simulink model "PubIfDecisionLM_MDL"  (R2020b)
settings: configuration reference "DspaceConfig" (kept outside this file)
PostLoadFcn:
  | if any(exist('dsrtsu_mdlpostloadfcn', 'file') ~= 0), dsrtsu_mdlpostloadfcn('Execute', bdroot); end
InitFcn:
  | , if any(exist('dsmpb_private', 'file') ~= 0), dsmpb_private('dsmpb_mdlclblib', 'Init', bdroot); end,
undefined symbols (not defined in the file or in its folder): OFM_OBJ_FUSIONTYPE_E, OFM_OBJ_MOVINGSTATE_E, OFM_OBJ_ORIENTATION_E, OFM_OBJ_TYPE_E, P_LM_Cyc, P_LM_EMLHistKapRcdBufSize, P_LM_EMLHistTrajBaseDis, P_LM_EMLHistTrajPNum, P_LM_EMLKapCorrMaxThre, P_LM_EMLMinKapThre, P_LM_EMLPathDisDiffThre, P_LM_EMLQuaFiltPar, P_LM_EMLTurnActKapThre, P_LM_EMLValidQuaThre, P_LM_FntPath1Disgap, P_LM_FntPath1MinDis, P_LM_FntPath1Timegap, P_LM_FntPath2Disgap, P_LM_FntPath2MinDis, P_LM_FntPath2Timegap, P_LM_FntPath3Disgap, P_LM_FntPath3MinDis, P_LM_FntPath3Timegap, P_LM_FusBLParFiltP, P_LM_FusEVDifC2Thre, P_LM_FusEVOPath1AllVSLDisThre, P_LM_FusEVOPath1AllVSLLostNumThre, P_LM_FusEVOPath1AllVSLQuaThre, P_LM_FusEVOPath1OTLFacNLC, P_LM_FusOTLQuaThre, P_LM_FusOTLSW, P_LM_FusParC0Index, P_LM_FusParC1Index, P_LM_FusParC2Index, P_LM_FusParC3Index, P_LM_FusVSLQuaThre, P_LM_FusVSLSW, P_LM_FusVSLValidSteerWheerAngThre, P_LM_FusVSLValidVxvThre, P_LM_LaneWidth, P_LM_OTLBufTPInfoEvaFactor, P_LM_OTLObjNum, P_LM_OTLObjSelectAgeThre, P_LM_OTLObjSelectDxAssessVx, P_LM_OTLObjSelectDxThre, P_LM_OTLObjSelectVxThre, P_LM_OTLObjSelectVyAssessDx, P_LM_OTLObjSelectVyThre, P_LM_OTLTrajPntBaseDis, P_LM_OTLTrajStdThre, P_LM_VSLAvailLineNum, P_LM_VSLBLSDiffThre, P_LM_VSLBLSDisRatio, P_LM_VSLFusBLParFiltP_C1, P_LM_VSLFusBLParFiltP_C2, P_LM_VSLFusBLParFiltP_C3, P_LM_VSLFusBLParFiltP_Quality, P_LM_VSLHistTrajBaseDis, P_LM_VSLHistTrajPNum, P_LM_VSLLCC0diff ... (+18)
libraries: simulink x145, LM_LIB x43
(part 7 of 24)

== system PubIfDecisionLM_MDL/Subsystem2/LM_EML/LM_EMLFntPath1/LM_EML_C0/Switch Case Action Subsystem1 ==
  P_LM_LaneWidth : Inport
  Action Port : ActionPort  ActionPortLabel=case [ 1 ]:
  Constant : Constant  Value=2  OutDataTypeStr=single
  Constant1 : Constant  Value=-1  OutDataTypeStr=single
  Divide : Product  Inputs=*/
  Product : Product
  Subtract : Sum  Inputs=+-
  Subtract1 : Sum  Inputs=+-
  LM_EML_LLC0 : Outport
  LM_EML_LRC0 : Outport  Port=2
  LM_EML_RLC0 : Outport  Port=3
  LM_EML_RRC0 : Outport  Port=4
  wires:
  Product/1 -> LM_EML_LRC0/1, Subtract1/1  "LM_EML_LRC0"
  Subtract/1 -> LM_EML_RRC0/1  "LM_EML_RRC0"
  P_LM_LaneWidth/1 -> Divide/1, Subtract/2, Subtract1/2
  Constant/1 -> Divide/2
  Subtract1/1 -> LM_EML_RLC0/1, Subtract/1  "LM_EML_RLC0"
  Constant1/1 -> Product/2
  Divide/1 -> LM_EML_LLC0/1, Product/1  "LM_EML_LRC0"

== system PubIfDecisionLM_MDL/Subsystem2/LM_EML/LM_EMLFntPath1/LM_EML_C0/Switch Case Action Subsystem2 ==
  P_LM_LaneWidth : Inport
  Action Port : ActionPort  ActionPortLabel=case [ 3 ]:
  Add : Sum
  Add1 : Sum
  Constant : Constant  Value=2  OutDataTypeStr=single
  Constant1 : Constant  Value=-1  OutDataTypeStr=single
  Divide : Product  Inputs=*/
  Product : Product
  LM_EML_LLC0 : Outport
  LM_EML_LRC0 : Outport  Port=2
  LM_EML_RLC0 : Outport  Port=3
  LM_EML_RRC0 : Outport  Port=4
  wires:
  Add/1 -> LM_EML_LRC0/1, Add1/2  "LM_EML_LRC0"
  Divide/1 -> LM_EML_RLC0/1, Add/2, Product/1  "LM_EML_RLC0"
  Constant1/1 -> Product/2
  Constant/1 -> Divide/2
  P_LM_LaneWidth/1 -> Add1/1, Add/1, Divide/1
  Add1/1 -> LM_EML_LLC0/1  "LM_EML_LLC0"
  Product/1 -> LM_EML_RRC0/1  "LM_EML_RRC0"

== system PubIfDecisionLM_MDL/Subsystem2/LM_EML/LM_EMLRearPath1/LM_EMLHistTrajCoordinateConvert/If Action Subsystem ==
  LM_ComEVOffsetX : Inport
  LM_ComEVOffsetY : Inport  Port=2
  LM_ComEVOffsetAng : Inport  Port=3
  LM_EMLHistTrajVectXK1 : Inport  Port=4
  LM_EMLHistTrajVectYK1 : Inport  Port=5
  Action Port : ActionPort  ActionPortLabel=if(u1 == 0)
  For Each Subsystem : Subsystem  TreatAsAtomicUnit=on
  LM_EMLHistTrajVectXK1Adju : Outport
  LM_EMLHistTrajVectYK1Adju : Outport  Port=2
  wires:
  For Each Subsystem/2(LM_EMLHistTrajVectYK1Adju) -> LM_EMLHistTrajVectYK1Adju/1
  For Each Subsystem/1(LM_EMLHistTrajVectXK1Adju) -> LM_EMLHistTrajVectXK1Adju/1
  LM_EMLHistTrajVectYK1/1 -> For Each Subsystem/5(LM_EMLHistTrajVectYK1)
  LM_EMLHistTrajVectXK1/1 -> For Each Subsystem/4(LM_EMLHistTrajVectXK1)
  LM_ComEVOffsetAng/1 -> For Each Subsystem/3(LM_ComEVOffsetAng)
  LM_ComEVOffsetY/1 -> For Each Subsystem/2(LM_ComEVOffsetY)
  LM_ComEVOffsetX/1 -> For Each Subsystem/1(LM_ComEVOffsetX)

== system PubIfDecisionLM_MDL/Subsystem2/LM_EML/LM_EMLRearPath1/LM_EMLHistTrajCoordinateConvert/If Action Subsystem1 ==
  LM_EMLHistTrajVectXK1 : Inport
  LM_EMLHistTrajVectYK1 : Inport  Port=2
  Action Port : ActionPort  ActionPortLabel=else
  LM_EMLHistTrajVectXK1Adju : Outport
  LM_EMLHistTrajVectYK1Adju : Outport  Port=2
  wires:
  LM_EMLHistTrajVectYK1/1 -> LM_EMLHistTrajVectYK1Adju/1
  LM_EMLHistTrajVectXK1/1 -> LM_EMLHistTrajVectXK1Adju/1

== system PubIfDecisionLM_MDL/Subsystem2/LM_Fusion1/LM_FusBaseLineFilt/LM_FusBaseLineInfoFilt/LM_FusBLFntPath1InfoFilt ==
  LM_FusBLPathC0 : Inport
  LM_FusBLPathC1 : Inport  Port=2
  LM_FusBLPathC2 : Inport  Port=3
  LM_FusBLPathC3 : Inport  Port=4
  LM_FusBLPathQuality : Inport  Port=5
  LM_FusBLPathQuliatyFilt : Subsystem
  LM_Fus_BLFntPathC0Filt : Subsystem
  LM_Fus_BLPath3C3Filt : Subsystem
  LM_Fus_BLPathC1Filt : Subsystem
  LM_Fus_BLPathC2Filt : Subsystem
  Unit Delay{,1..4} (5 alike) : UnitDelay  SampleTime=-1  HasFrameUpgradeWarning=on
  LM_FusBLPathC0Filt : Outport
  LM_FusBLPathC1Filt : Outport  Port=2
  LM_FusBLPathC2Filt : Outport  Port=3
  LM_FusBLPathC3Filt : Outport  Port=4
  LM_FusBLPathQualityFilt : Outport  Port=5
  wires:
  LM_Fus_BLPathC1Filt/1(LM_FusBLPathC1Filt) -> Unit Delay1/1, LM_FusBLPathC1Filt/1
  LM_Fus_BLFntPathC0Filt/1(LM_FusBLPathC0Filt) -> Unit Delay/1, LM_FusBLPathC0Filt/1
  LM_FusBLPathC0/1 -> LM_Fus_BLFntPathC0Filt/1(LM_FusBLPathC0)
  LM_FusBLPathQuality/1 -> LM_FusBLPathQuliatyFilt/1(LM_FusBLPathQuality), LM_Fus_BLPath3C3Filt/2(LM_FusBLPathQuality), LM_Fus_BLPathC2Filt/2(LM_FusBLPathQuality), LM_Fus_BLPathC1Filt/2(LM_FusBLPathQuality), LM_Fus_BLFntPathC0Filt/2(LM_FusBLPathQuality)
  Unit Delay/1 -> LM_Fus_BLFntPathC0Filt/4(LM_FusBLPathC0K1)
  LM_FusBLPathC1/1 -> LM_Fus_BLPathC1Filt/3(LM_FusBLPathC1BefFilt)
  Unit Delay1/1 -> LM_Fus_BLPathC1Filt/4(LM_FusBLPathC1K1)
  LM_FusBLPathC2/1 -> LM_Fus_BLPathC2Filt/3(LM_FusBLPathC2BefFilt)
  Unit Delay2/1 -> LM_Fus_BLPathC2Filt/4(LM_FusBLPathC2K1)
  LM_Fus_BLPathC2Filt/1(LM_FusBLPathC2Filt) -> LM_FusBLPathC2Filt/1, Unit Delay2/1
  LM_FusBLPathC3/1 -> LM_Fus_BLPath3C3Filt/3(LM_FusBLPathC3BefFilt)
  Unit Delay3/1 -> LM_Fus_BLPath3C3Filt/4(LM_FusBLPathC3K1)
  LM_Fus_BLPath3C3Filt/1(LM_FusBLPathC3Filt) -> LM_FusBLPathC3Filt/1, Unit Delay3/1
  LM_FusBLPathQuliatyFilt/1(LM_FusBLPathQualityFilt) -> LM_FusBLPathQualityFilt/1, Unit Delay4/1
  Unit Delay4/1 -> LM_Fus_BLPath3C3Filt/1(LM_FusBLPathQualityK1), LM_Fus_BLPathC2Filt/1(LM_FusBLPathQualityK1), LM_Fus_BLPathC1Filt/1(LM_FusBLPathQualityK1), LM_Fus_BLFntPathC0Filt/3(LM_FusBLPathQualityK1), LM_FusBLPathQuliatyFilt/2(LM_FusBLPathQualityK1)

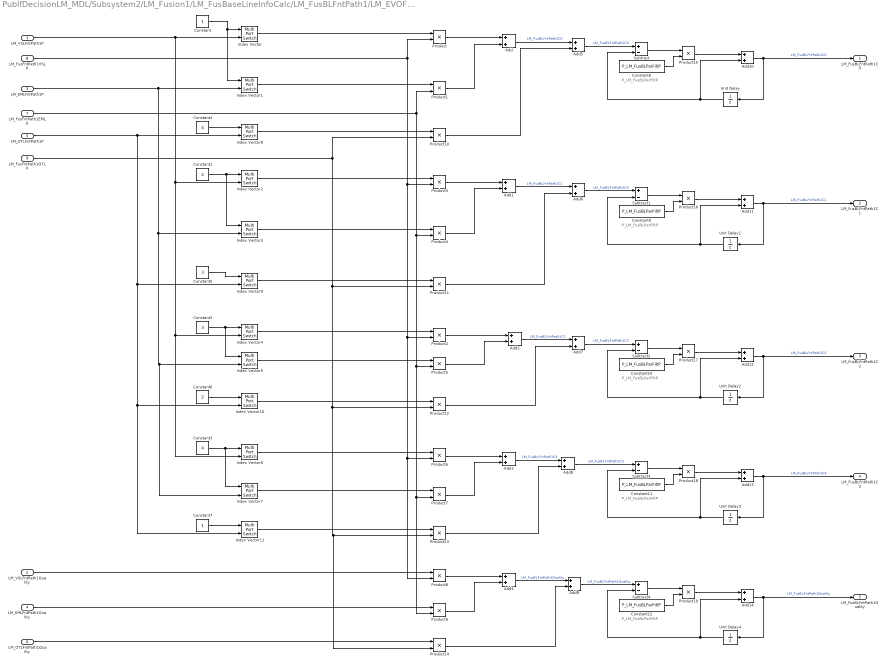
== system PubIfDecisionLM_MDL/Subsystem2/LM_Fusion1/LM_FusBaseLineInfoCalc/LM_FusBLFntPath1/LM_EVOFFntPath1 ==
  note: P_LM_FusBLParFiltP
  note: P_LM_FusBLParFiltP
  note: P_LM_FusBLParFiltP
  note: P_LM_FusBLParFiltP
  note: P_LM_FusBLParFiltP
  LM_VSLFntPath1P : Inport
  LM_VSLFntPath1Quality : Inport  Port=2
  LM_EMLFntPath1P : Inport  Port=3
  LM_EMLFntPath1Quality : Inport  Port=4
  LM_OTLFntPath1P : Inport  Port=5
  LM_OTLFntPath1Quality : Inport  Port=6
  LM_FusFntPath1EMLK : Inport  Port=7
  LM_FusFntPath1VSLK : Inport  Port=8
  LM_FusFntPath1OTLK : Inport  Port=9
  Add{,1..14} (15 alike) : Sum
  Constant : Constant  OutDataTypeStr=uint8
  Constant1 : Constant  Value=2  OutDataTypeStr=uint8
  Constant{8..12} (5 alike) : Constant  Value=P_LM_FusBLParFiltP  OutDataTypeStr=single
  Constant2 : Constant  Value=3  OutDataTypeStr=uint8
  Constant3 : Constant  Value=4  OutDataTypeStr=uint8
  Constant4 : Constant  Value=4  OutDataTypeStr=uint8
  Constant5 : Constant  Value=3  OutDataTypeStr=uint8
  Constant6 : Constant  Value=2  OutDataTypeStr=uint8
  Constant7 : Constant  OutDataTypeStr=uint8
  Index Vector{,1..11} (12 alike) : MultiPortSwitch  Inputs=1
  Product{,1..19} (20 alike) : Product
  Subtract{,1..4} (5 alike) : Sum  Inputs=+-
  Unit Delay{,1..4} (5 alike) : UnitDelay  SampleTime=-1  HasFrameUpgradeWarning=on
  LM_FusBLFntPath1C0 : Outport
  LM_FusBLFntPath1C1 : Outport  Port=2
  LM_FusBLFntPath1C2 : Outport  Port=3
  LM_FusBLFntPath1C3 : Outport  Port=4
  LM_FusBLFntPath1Quality : Outport  Port=5
  wires:
  LM_VSLFntPath1Quality/1 -> Product8/1
  Add9/1 -> Subtract4/1  "LM_FusBLFntPath1Quality"
  Constant12/1 -> Product19/2
  Subtract4/1 -> Product19/1
  Product19/1 -> Add14/1
  Unit Delay4/1 -> Subtract4/2, Add14/2
  Add8/1 -> Subtract3/1  "LM_FusBLFntPath1C3"
  Unit Delay3/1 -> Add13/2, Subtract3/2
  Product18/1 -> Add13/1
  Subtract3/1 -> Product18/1
  Constant11/1 -> Product18/2
  Add7/1 -> Subtract2/1  "LM_FusBLFntPath1C2"
  Constant10/1 -> Product17/2
  Subtract2/1 -> Product17/1
  Product17/1 -> Add12/1
  Unit Delay2/1 -> Subtract2/2, Add12/2
  Add6/1 -> Subtract1/1  "LM_FusBLFntPath1C0"
  Unit Delay1/1 -> Add11/2, Subtract1/2
  Product16/1 -> Add11/1
  Subtract1/1 -> Product16/1
  Constant9/1 -> Product16/2
  Constant8/1 -> Product15/2
  Subtract/1 -> Product15/1
  Product15/1 -> Add10/1
  Unit Delay/1 -> Subtract/2, Add10/2
  Add5/1 -> Subtract/1  "LM_FusBLFntPath1C0"
  Constant7/1 -> Index Vector11/1
  Constant6/1 -> Index Vector10/1
  Constant5/1 -> Index Vector9/1
  Constant4/1 -> Index Vector8/1
  Product14/1 -> Add9/2
  Add4/1 -> Add9/1  "LM_FusBLFntPath1Quality"
  LM_OTLFntPath1Quality/1 -> Product14/1
  Product13/1 -> Add8/2
  Add3/1 -> Add8/1  "LM_FusBLFntPath1C3"
  Index Vector11/1 -> Product13/1
  Product12/1 -> Add7/2
  Add2/1 -> Add7/1  "LM_FusBLFntPath1C2"
  Index Vector10/1 -> Product12/1
  Product11/1 -> Add6/2
  Add1/1 -> Add6/1  "LM_FusBLFntPath1C1"
  Index Vector9/1 -> Product11/1
  Product10/1 -> Add5/2
  Add/1 -> Add5/1  "LM_FusBLFntPath1C0"
  LM_FusFntPath1OTLK/1 -> Product10/2, Product11/2, Product12/2, Product13/2, Product14/2
  Index Vector8/1 -> Product10/1
  LM_OTLFntPath1P/1 -> Index Vector8/2, Index Vector9/2, Index Vector10/2, Index Vector11/2
  Constant3/1 -> Index Vector6/1, Index Vector7/1
  Constant2/1 -> Index Vector4/1, Index Vector5/1
  Constant1/1 -> Index Vector2/1, Index Vector3/1
  Constant/1 -> Index Vector/1, Index Vector1/1
  LM_VSLFntPath1P/1 -> Index Vector2/2, Index Vector4/2, Index Vector6/2, Index Vector/2
  Add14/1 -> Unit Delay4/1, LM_FusBLFntPath1Quality/1  "LM_FusBLFntPath1Quality"
  Product9/1 -> Add4/2
  Product8/1 -> Add4/1
  LM_EMLFntPath1Quality/1 -> Product9/1
  Add13/1 -> Unit Delay3/1, LM_FusBLFntPath1C3/1  "LM_FusBLFntPath1C3"
  Product7/1 -> Add3/2
  Product6/1 -> Add3/1
  Index Vector7/1 -> Product7/1
  Index Vector6/1 -> Product6/1
  LM_EMLFntPath1P/1 -> Index Vector1/2, Index Vector3/2, Index Vector5/2, Index Vector7/2
  Index Vector/1 -> Product/1
  Product5/1 -> Add2/2
  LM_FusFntPath1EMLK/1 -> Product4/2, Product7/2, Product9/2, Product5/2, Product1/2
  Index Vector5/1 -> Product5/1
  Product2/1 -> Add2/1
  LM_FusFntPath1VSLK/1 -> Product3/2, Product6/2, Product8/2, Product2/2, Product/2
  Index Vector4/1 -> Product2/1
  Index Vector2/1 -> Product3/1
  Product3/1 -> Add1/1
  Index Vector3/1 -> Product4/1
  Product4/1 -> Add1/2
  Product1/1 -> Add/2
  Index Vector1/1 -> Product1/1
  Product/1 -> Add/1
  Add12/1 -> Unit Delay2/1, LM_FusBLFntPath1C2/1  "LM_FusBLFntPath1C2"
  Add11/1 -> Unit Delay1/1, LM_FusBLFntPath1C1/1  "LM_FusBLFntPath1C1"
  Add10/1 -> LM_FusBLFntPath1C0/1, Unit Delay/1  "LM_FusBLFntPath1C0"

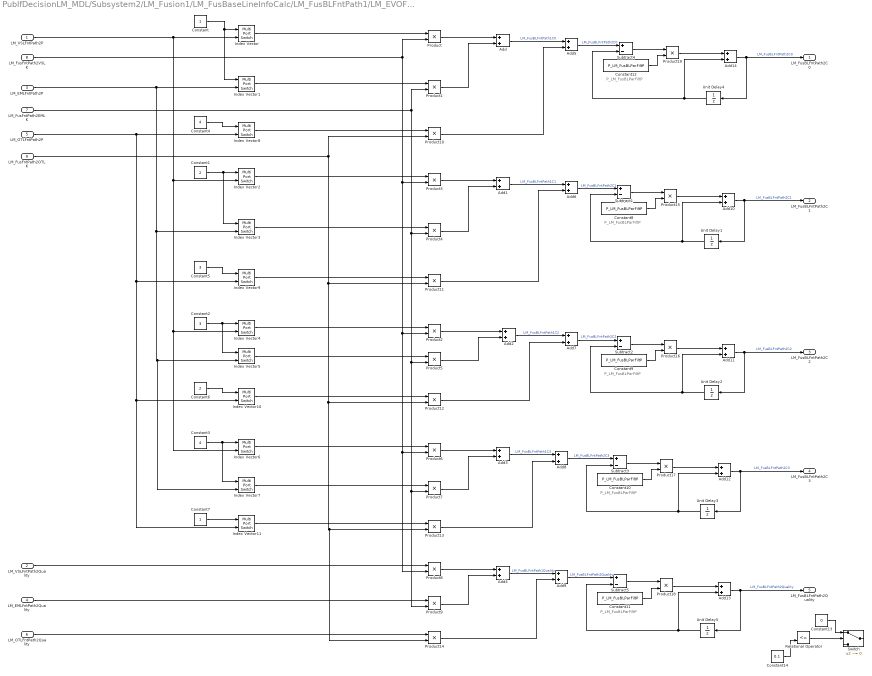
== system PubIfDecisionLM_MDL/Subsystem2/LM_Fusion1/LM_FusBaseLineInfoCalc/LM_FusBLFntPath1/LM_EVOFFntPath2 ==
  note: P_LM_FusBLParFiltP
  note: P_LM_FusBLParFiltP
  note: P_LM_FusBLParFiltP
  note: P_LM_FusBLParFiltP
  note: P_LM_FusBLParFiltP
  LM_VSLFntPath2P : Inport
  LM_VSLFntPath2Quality : Inport  Port=2
  LM_EMLFntPath2P : Inport  Port=3
  LM_EMLFntPath2Quality : Inport  Port=4
  LM_OTLFntPath2P : Inport  Port=5
  LM_OTLFntPath2Quality : Inport  Port=6
  LM_FusFntPath2EMLK : Inport  Port=7
  LM_FusFntPath2VSLK : Inport  Port=8
  LM_FusFntPath2OTLK : Inport  Port=9
  Add{,1..14} (15 alike) : Sum
  Constant : Constant  OutDataTypeStr=uint8
  Constant1 : Constant  Value=2  OutDataTypeStr=uint8
  Constant{8..12} (5 alike) : Constant  Value=P_LM_FusBLParFiltP  OutDataTypeStr=single
  Constant13 : Constant  Value=0  OutDataTypeStr=single
  Constant14 : Constant  Value=0.1  OutDataTypeStr=single
  Constant2 : Constant  Value=3  OutDataTypeStr=uint8
  Constant3 : Constant  Value=4  OutDataTypeStr=uint8
  Constant4 : Constant  Value=4  OutDataTypeStr=uint8
  Constant5 : Constant  Value=3  OutDataTypeStr=uint8
  Constant6 : Constant  Value=2  OutDataTypeStr=uint8
  Constant7 : Constant  OutDataTypeStr=uint8
  Index Vector{,1..11} (12 alike) : MultiPortSwitch  Inputs=1
  Product{,1..19} (20 alike) : Product
  Relational Operator : RelationalOperator  Operator=<=  OutDataTypeStr=boolean  RndMeth=Simplest
  Subtract{1..5} (5 alike) : Sum  Inputs=+-
  Switch : Switch  Criteria=u2 ~= 0
  Unit Delay{1..5} (5 alike) : UnitDelay  SampleTime=-1  HasFrameUpgradeWarning=on
  LM_FusBLFntPath2C0 : Outport
  LM_FusBLFntPath2C1 : Outport  Port=2
  LM_FusBLFntPath2C2 : Outport  Port=3
  LM_FusBLFntPath2C3 : Outport  Port=4
  LM_FusBLFntPath2Quality : Outport  Port=5
  wires:
  Relational Operator/1 -> Switch/2
  ? -> Relational Operator/1, Switch/3
  Constant14/1 -> Relational Operator/2
  Constant13/1 -> Switch/1
  Add9/1 -> Subtract5/1  "LM_FusBLFntPath2Quality"
  Constant11/1 -> Product18/2
  Unit Delay5/1 -> Subtract5/2, Add13/2
  Product18/1 -> Add13/1
  Subtract5/1 -> Product18/1
  Add8/1 -> Subtract3/1  "LM_FusBLFntPath2C3"
  Constant10/1 -> Product17/2
  Unit Delay3/1 -> Subtract3/2, Add12/2
  Product17/1 -> Add12/1
  Subtract3/1 -> Product17/1
  Add7/1 -> Subtract2/1  "LM_FusBLFntPath2C2"
  Constant9/1 -> Product16/2
  Unit Delay2/1 -> Subtract2/2, Add11/2
  Product16/1 -> Add11/1
  Subtract2/1 -> Product16/1
  Add6/1 -> Subtract1/1  "LM_FusBLFntPath2C1"
  Constant8/1 -> Product15/2
  Unit Delay1/1 -> Subtract1/2, Add10/2
  Product15/1 -> Add10/1
  Subtract1/1 -> Product15/1
  Add5/1 -> Subtract4/1  "LM_FusBLFntPath2C0"
  Constant12/1 -> Product19/2
  Unit Delay4/1 -> Subtract4/2, Add14/2
  Product19/1 -> Add14/1
  Subtract4/1 -> Product19/1
  Constant7/1 -> Index Vector11/1
  Constant6/1 -> Index Vector10/1
  Constant5/1 -> Index Vector9/1
  Constant4/1 -> Index Vector8/1
  Add14/1 -> Unit Delay4/1, LM_FusBLFntPath2C0/1  "LM_FusBLFntPath2C0"
  Add10/1 -> Unit Delay1/1, LM_FusBLFntPath2C1/1  "LM_FusBLFntPath2C1"
  Add11/1 -> Unit Delay2/1, LM_FusBLFntPath2C2/1  "LM_FusBLFntPath2C2"
  Product/1 -> Add/1
  Index Vector1/1 -> Product1/1
  Product1/1 -> Add/2
  Product4/1 -> Add1/2
  Index Vector3/1 -> Product4/1
  Product3/1 -> Add1/1
  Index Vector2/1 -> Product3/1
  Index Vector4/1 -> Product2/1
  LM_FusFntPath2VSLK/1 -> Product/2, Product2/2, Product8/2, Product6/2, Product3/2
  Product2/1 -> Add2/1
  Index Vector5/1 -> Product5/1
  LM_FusFntPath2EMLK/1 -> Product1/2, Product5/2, Product9/2, Product7/2, Product4/2
  Product5/1 -> Add2/2
  Index Vector/1 -> Product/1
  LM_EMLFntPath2P/1 -> Index Vector7/2, Index Vector5/2, Index Vector3/2, Index Vector1/2
  Index Vector6/1 -> Product6/1
  Index Vector7/1 -> Product7/1
  Product6/1 -> Add3/1
  Product7/1 -> Add3/2
  Add12/1 -> Unit Delay3/1, LM_FusBLFntPath2C3/1  "LM_FusBLFntPath2C3"
  LM_VSLFntPath2Quality/1 -> Product8/1
  LM_EMLFntPath2Quality/1 -> Product9/1
  Product8/1 -> Add4/1
  Product9/1 -> Add4/2
  Add13/1 -> Unit Delay5/1, LM_FusBLFntPath2Quality/1  "LM_FusBLFntPath2Quality"
  LM_VSLFntPath2P/1 -> Index Vector/2, Index Vector6/2, Index Vector4/2, Index Vector2/2
  Constant/1 -> Index Vector1/1, Index Vector/1
  Constant1/1 -> Index Vector3/1, Index Vector2/1
  Constant2/1 -> Index Vector5/1, Index Vector4/1
  Constant3/1 -> Index Vector7/1, Index Vector6/1
  LM_OTLFntPath2P/1 -> Index Vector11/2, Index Vector10/2, Index Vector9/2, Index Vector8/2
  Index Vector8/1 -> Product10/1
  LM_FusFntPath2OTLK/1 -> Product14/2, Product13/2, Product12/2, Product11/2, Product10/2
  Add/1 -> Add5/1  "LM_FusBLFntPath1C0"
  Product10/1 -> Add5/2
  Index Vector9/1 -> Product11/1
  Add1/1 -> Add6/1  "LM_FusBLFntPath1C1"
  Product11/1 -> Add6/2
  Index Vector10/1 -> Product12/1
  Add2/1 -> Add7/1  "LM_FusBLFntPath1C2"
  Product12/1 -> Add7/2
  Index Vector11/1 -> Product13/1
  Add3/1 -> Add8/1  "LM_FusBLFntPath1C3"
  Product13/1 -> Add8/2
  LM_OTLFntPath2Quality/1 -> Product14/1
  Add4/1 -> Add9/1  "LM_FusBLFntPath1Quality"
  Product14/1 -> Add9/2

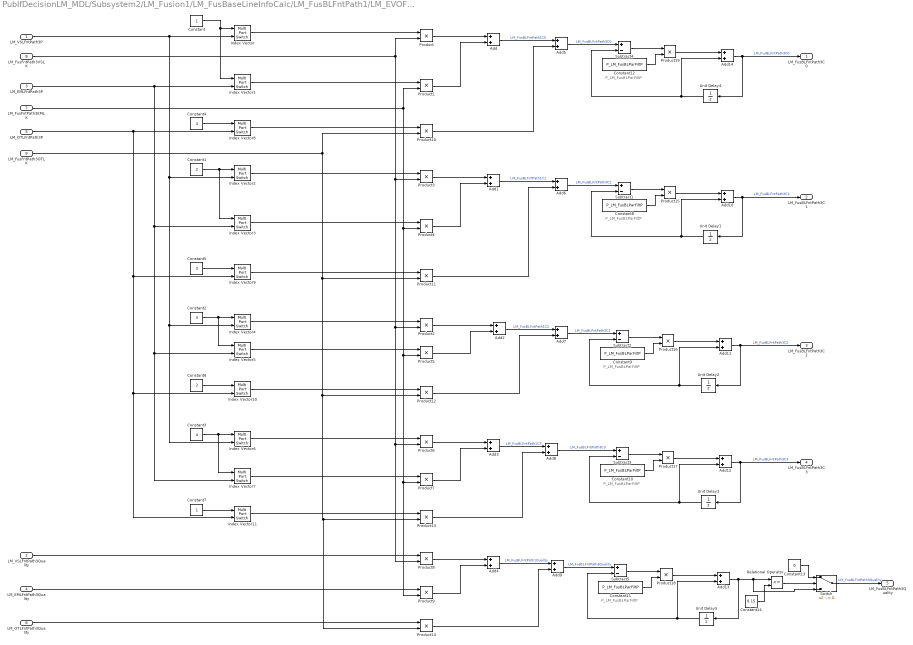
== system PubIfDecisionLM_MDL/Subsystem2/LM_Fusion1/LM_FusBaseLineInfoCalc/LM_FusBLFntPath1/LM_EVOFFntPath3 ==
  note: P_LM_FusBLParFiltP
  note: P_LM_FusBLParFiltP
  note: P_LM_FusBLParFiltP
  note: P_LM_FusBLParFiltP
  note: P_LM_FusBLParFiltP
  LM_VSLFntPath3P : Inport
  LM_VSLFntPath3Quality : Inport  Port=2
  LM_EMLFntPath3P : Inport  Port=3
  LM_EMLFntPath3Quality : Inport  Port=4
  LM_OTLFntPath3P : Inport  Port=5
  LM_OTLFntPath3Quality : Inport  Port=6
  LM_FusFntPath3EMLK : Inport  Port=7
  LM_FusFntPath3VSLK : Inport  Port=8
  LM_FusFntPath3OTLK : Inport  Port=9
  Add{,1..14} (15 alike) : Sum
  Constant : Constant  OutDataTypeStr=uint8
  Constant1 : Constant  Value=2  OutDataTypeStr=uint8
  Constant{8..12} (5 alike) : Constant  Value=P_LM_FusBLParFiltP  OutDataTypeStr=single
  Constant13 : Constant  Value=0  OutDataTypeStr=single
  Constant14 : Constant  Value=0.15  OutDataTypeStr=single
  Constant2 : Constant  Value=3  OutDataTypeStr=uint8
  Constant3 : Constant  Value=4  OutDataTypeStr=uint8
  Constant4 : Constant  Value=4  OutDataTypeStr=uint8
  Constant5 : Constant  Value=3  OutDataTypeStr=uint8
  Constant6 : Constant  Value=2  OutDataTypeStr=uint8
  Constant7 : Constant  OutDataTypeStr=uint8
  Index Vector{,1..11} (12 alike) : MultiPortSwitch  Inputs=1
  Product{,1..19} (20 alike) : Product
  Relational Operator : RelationalOperator  Operator=<=  OutDataTypeStr=boolean  RndMeth=Simplest
  Subtract{1..5} (5 alike) : Sum  Inputs=+-
  Switch : Switch  Criteria=u2 ~= 0
  Unit Delay{1..5} (5 alike) : UnitDelay  SampleTime=-1  HasFrameUpgradeWarning=on
  LM_FusBLFntPath3C0 : Outport
  LM_FusBLFntPath3C1 : Outport  Port=2
  LM_FusBLFntPath3C2 : Outport  Port=3
  LM_FusBLFntPath3C3 : Outport  Port=4
  LM_FusBLFntPath3Quality : Outport  Port=5
  wires:
  Switch/1 -> LM_FusBLFntPath3Quality/1  "LM_FusBLFntPath3Quality"
  Constant14/1 -> Relational Operator/2
  Constant13/1 -> Switch/1
  Relational Operator/1 -> Switch/2
  Add9/1 -> Subtract5/1  "LM_FusBLFntPath3Quality"
  Constant11/1 -> Product18/2
  Unit Delay5/1 -> Subtract5/2, Add13/2
  Product18/1 -> Add13/1
  Subtract5/1 -> Product18/1
  Add8/1 -> Subtract3/1  "LM_FusBLFntPath3C3"
  Constant10/1 -> Product17/2
  Unit Delay3/1 -> Subtract3/2, Add12/2
  Product17/1 -> Add12/1
  Subtract3/1 -> Product17/1
  Add7/1 -> Subtract2/1  "LM_FusBLFntPath3C2"
  Constant9/1 -> Product16/2
  Unit Delay2/1 -> Subtract2/2, Add11/2
  Product16/1 -> Add11/1
  Subtract2/1 -> Product16/1
  Add6/1 -> Subtract1/1  "LM_FusBLFntPath3C1"
  Constant8/1 -> Product15/2
  Unit Delay1/1 -> Subtract1/2, Add10/2
  Product15/1 -> Add10/1
  Subtract1/1 -> Product15/1
  Add5/1 -> Subtract4/1  "LM_FusBLFntPath3C0"
  Constant12/1 -> Product19/2
  Unit Delay4/1 -> Subtract4/2, Add14/2
  Product19/1 -> Add14/1
  Subtract4/1 -> Product19/1
  Constant7/1 -> Index Vector11/1
  Constant6/1 -> Index Vector10/1
  Constant5/1 -> Index Vector9/1
  Constant4/1 -> Index Vector8/1
  Product14/1 -> Add9/2
  Add4/1 -> Add9/1  "LM_FusBLFntPath1Quality"
  LM_OTLFntPath3Quality/1 -> Product14/1
  Product13/1 -> Add8/2
  Add3/1 -> Add8/1  "LM_FusBLFntPath1C3"
  Index Vector11/1 -> Product13/1
  Product12/1 -> Add7/2
  Add2/1 -> Add7/1  "LM_FusBLFntPath1C2"
  Index Vector10/1 -> Product12/1
  Product11/1 -> Add6/2
  Add1/1 -> Add6/1  "LM_FusBLFntPath1C1"
  Index Vector9/1 -> Product11/1
  Product10/1 -> Add5/2
  Add/1 -> Add5/1  "LM_FusBLFntPath1C0"
  LM_FusFntPath3OTLK/1 -> Product10/2, Product11/2, Product12/2, Product13/2, Product14/2
  Index Vector8/1 -> Product10/1
  LM_OTLFntPath3P/1 -> Index Vector8/2, Index Vector9/2, Index Vector10/2, Index Vector11/2
  Constant3/1 -> Index Vector6/1, Index Vector7/1
  Constant2/1 -> Index Vector4/1, Index Vector5/1
  Constant1/1 -> Index Vector2/1, Index Vector3/1
  Constant/1 -> Index Vector/1, Index Vector1/1
  LM_VSLFntPath3P/1 -> Index Vector2/2, Index Vector4/2, Index Vector6/2, Index Vector/2
  Add13/1 -> Unit Delay5/1, Relational Operator/1, Switch/3
  Product9/1 -> Add4/2
  Product8/1 -> Add4/1
  LM_EMLFntPath3Quality/1 -> Product9/1
  LM_VSLFntPath3Quality/1 -> Product8/1
  Add12/1 -> LM_FusBLFntPath3C3/1, Unit Delay3/1  "LM_FusBLFntPath3C3"
  Product7/1 -> Add3/2
  Product6/1 -> Add3/1
  Index Vector7/1 -> Product7/1
  Index Vector6/1 -> Product6/1
  LM_EMLFntPath3P/1 -> Index Vector1/2, Index Vector3/2, Index Vector5/2, Index Vector7/2
  Index Vector/1 -> Product/1
  Product5/1 -> Add2/2
  LM_FusFntPath3EMLK/1 -> Product4/2, Product7/2, Product9/2, Product5/2, Product1/2
  Index Vector5/1 -> Product5/1
  Product2/1 -> Add2/1
  LM_FusFntPath3VSLK/1 -> Product3/2, Product6/2, Product8/2, Product2/2, Product/2
  Index Vector4/1 -> Product2/1
  Index Vector2/1 -> Product3/1
  Product3/1 -> Add1/1
  Index Vector3/1 -> Product4/1
  Product4/1 -> Add1/2
  Product1/1 -> Add/2
  Index Vector1/1 -> Product1/1
  Product/1 -> Add/1
  Add11/1 -> Unit Delay2/1, LM_FusBLFntPath3C2/1  "LM_FusBLFntPath3C2"
  Add10/1 -> Unit Delay1/1, LM_FusBLFntPath3C1/1  "LM_FusBLFntPath3C1"
  Add14/1 -> Unit Delay4/1, LM_FusBLFntPath3C0/1  "LM_FusBLFntPath3C0"

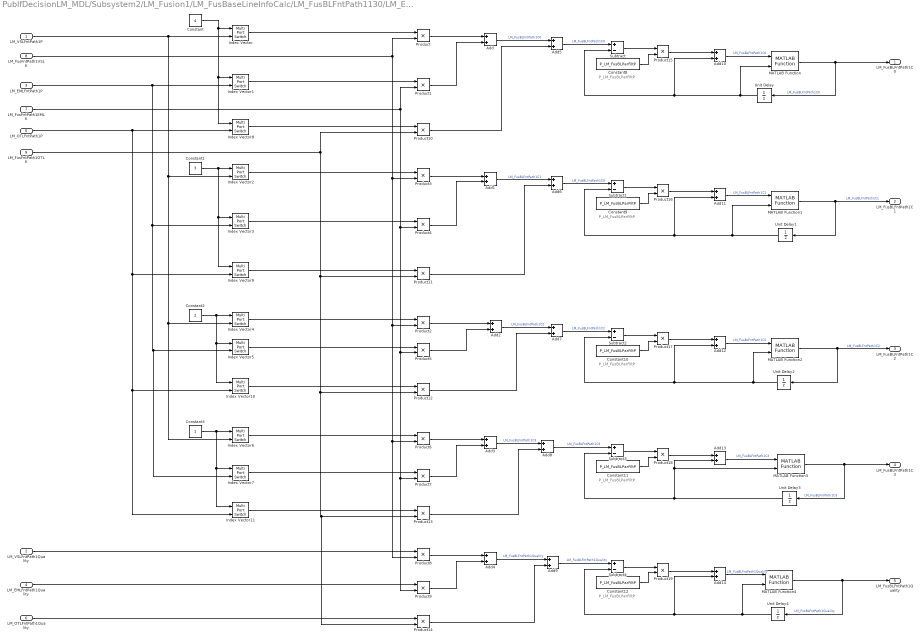
== system PubIfDecisionLM_MDL/Subsystem2/LM_Fusion1/LM_FusBaseLineInfoCalc/LM_FusBLFntPath1130/LM_EVOFFntPath1 ==
  note: P_LM_FusBLParFiltP
  note: P_LM_FusBLParFiltP
  note: P_LM_FusBLParFiltP
  note: P_LM_FusBLParFiltP
  note: P_LM_FusBLParFiltP
  LM_VSLFntPath1P : Inport
  LM_VSLFntPath1Quality : Inport  Port=2
  LM_EMLFntPath1P : Inport  Port=3
  LM_EMLFntPath1Quality : Inport  Port=4
  LM_OTLFntPath1P : Inport  Port=5
  LM_OTLFntPath1Quality : Inport  Port=6
  LM_FusFntPath1EMLK : Inport  Port=7
  LM_FusFntPath1VSLK : Inport  Port=8
  LM_FusFntPath1OTLK : Inport  Port=9
  Add{,1..14} (15 alike) : Sum
  Constant : Constant  Value=4  OutDataTypeStr=uint8
  Constant1 : Constant  Value=3  OutDataTypeStr=uint8
  Constant{8..12} (5 alike) : Constant  Value=P_LM_FusBLParFiltP  OutDataTypeStr=single
  Constant2 : Constant  Value=2  OutDataTypeStr=uint8
  Constant3 : Constant  OutDataTypeStr=uint8
  Index Vector{,1..11} (12 alike) : MultiPortSwitch  Inputs=1
  MATLAB Function{,1..4} (5 alike) : LM_LIB/LM_EVOFusPath/LM_FusBLPathQualityCalc/MATLAB Function  SystemSampleTime=-1  SSRTWFcnClass=[]  Latency=0  AutoFrameSizeCalculation=off
  Product{,1..19} (20 alike) : Product
  Subtract{,1..4} (5 alike) : Sum  Inputs=+-
  Unit Delay{,1..4} (5 alike) : UnitDelay  SampleTime=-1  HasFrameUpgradeWarning=on
  LM_FusBLFntPath1C0 : Outport
  LM_FusBLFntPath1C1 : Outport  Port=2
  LM_FusBLFntPath1C2 : Outport  Port=3
  LM_FusBLFntPath1C3 : Outport  Port=4
  LM_FusBLFntPath1Quality : Outport  Port=5
  wires:
  Add14/1 -> MATLAB Function4/1  "LM_FusBLFntPath1Quality"
  Add13/1 -> MATLAB Function3/1  "LM_FusBLFntPath1C3"
  Add12/1 -> MATLAB Function2/1  "LM_FusBLFntPath1C2"
  Add11/1 -> MATLAB Function1/1  "LM_FusBLFntPath1C1"
  Unit Delay/1 -> Add10/2, Subtract/2, MATLAB Function/2
  Add10/1 -> MATLAB Function/1  "LM_FusBLFntPath1C0"
  MATLAB Function/1 -> Unit Delay/1, LM_FusBLFntPath1C0/1  "LM_FusBLFntPath1C0"
  MATLAB Function1/1 -> Unit Delay1/1, LM_FusBLFntPath1C1/1  "LM_FusBLFntPath1C1"
  MATLAB Function2/1 -> LM_FusBLFntPath1C2/1, Unit Delay2/1  "LM_FusBLFntPath1C2"
  Product/1 -> Add/1
  Index Vector1/1 -> Product1/1
  Product1/1 -> Add/2
  Product4/1 -> Add1/2
  Index Vector3/1 -> Product4/1
  Product3/1 -> Add1/1
  Index Vector2/1 -> Product3/1
  Index Vector4/1 -> Product2/1
  LM_FusFntPath1VSLK/1 -> Product/2, Product2/2, Product8/2, Product6/2, Product3/2
  Product2/1 -> Add2/1
  Index Vector5/1 -> Product5/1
  LM_FusFntPath1EMLK/1 -> Product1/2, Product5/2, Product9/2, Product7/2, Product4/2
  Product5/1 -> Add2/2
  Index Vector/1 -> Product/1
  LM_EMLFntPath1P/1 -> Index Vector7/2, Index Vector5/2, Index Vector3/2, Index Vector1/2
  Index Vector6/1 -> Product6/1
  Index Vector7/1 -> Product7/1
  Product6/1 -> Add3/1
  Product7/1 -> Add3/2
  MATLAB Function3/1 -> LM_FusBLFntPath1C3/1, Unit Delay3/1  "LM_FusBLFntPath1C3"
  LM_EMLFntPath1Quality/1 -> Product9/1
  Product8/1 -> Add4/1
  Product9/1 -> Add4/2
  MATLAB Function4/1 -> LM_FusBLFntPath1Quality/1, Unit Delay4/1  "LM_FusBLFntPath1Quality"
  LM_VSLFntPath1P/1 -> Index Vector/2, Index Vector6/2, Index Vector4/2, Index Vector2/2
  LM_OTLFntPath1P/1 -> Index Vector11/2, Index Vector10/2, Index Vector9/2, Index Vector8/2
  Index Vector8/1 -> Product10/1
  LM_FusFntPath1OTLK/1 -> Product14/2, Product13/2, Product12/2, Product11/2, Product10/2
  Add/1 -> Add5/1  "LM_FusBLFntPath1C0"
  Product10/1 -> Add5/2
  Index Vector9/1 -> Product11/1
  Add1/1 -> Add6/1  "LM_FusBLFntPath1C1"
  Product11/1 -> Add6/2
  Index Vector10/1 -> Product12/1
  Add2/1 -> Add7/1  "LM_FusBLFntPath1C2"
  Product12/1 -> Add7/2
  Index Vector11/1 -> Product13/1
  Add3/1 -> Add8/1  "LM_FusBLFntPath1C3"
  Product13/1 -> Add8/2
  LM_OTLFntPath1Quality/1 -> Product14/1
  Add4/1 -> Add9/1  "LM_FusBLFntPath1Quality"
  Product14/1 -> Add9/2
  Constant/1 -> Index Vector1/1, Index Vector8/1, Index Vector/1
  Constant1/1 -> Index Vector3/1, Index Vector9/1, Index Vector2/1
  Constant2/1 -> Index Vector5/1, Index Vector10/1, Index Vector4/1
  Constant3/1 -> Index Vector7/1, Index Vector11/1, Index Vector6/1
  Add5/1 -> Subtract/1  "LM_FusBLFntPath1C0"
  Product15/1 -> Add10/1
  Subtract/1 -> Product15/1
  Constant8/1 -> Product15/2
  Constant9/1 -> Product16/2
  Subtract1/1 -> Product16/1
  Product16/1 -> Add11/1
  Unit Delay1/1 -> Subtract1/2, Add11/2, MATLAB Function1/2
  Add6/1 -> Subtract1/1  "LM_FusBLFntPath1C0"
  Unit Delay2/1 -> Add12/2, Subtract2/2, MATLAB Function2/2
  Product17/1 -> Add12/1
  Subtract2/1 -> Product17/1
  Constant10/1 -> Product17/2
  Add7/1 -> Subtract2/1  "LM_FusBLFntPath1C2"
  Constant11/1 -> Product18/2
  Subtract3/1 -> Product18/1
  Product18/1 -> Add13/1
  Unit Delay3/1 -> Subtract3/2, Add13/2, MATLAB Function3/2
  Add8/1 -> Subtract3/1  "LM_FusBLFntPath1C3"
  Unit Delay4/1 -> Add14/2, Subtract4/2, MATLAB Function4/2
  Product19/1 -> Add14/1
  Subtract4/1 -> Product19/1
  Constant12/1 -> Product19/2
  Add9/1 -> Subtract4/1  "LM_FusBLFntPath1Quality"
  LM_VSLFntPath1Quality/1 -> Product8/1

== system PubIfDecisionLM_MDL/Subsystem2/LM_Fusion1/LM_FusBaseLineInfoCalc/LM_FusBLFntPath1130/LM_EVOFFntPath2 ==
  LM_VSLFntPathP : Inport
  LM_VSLPathQuality : Inport  Port=2
  LM_EMLFntPathP : Inport  Port=3
  LM_EMLPathQuality : Inport  Port=4
  LM_OTLFntPathP : Inport  Port=5
  LM_OTLPathQuality : Inport  Port=6
  LM_FusPathEMLK : Inport  Port=7
  LM_FusPathVSLK : Inport  Port=8
  LM_FusPathOTLK : Inport  Port=9
  LM_FusBLPathC0Calc : Subsystem
  LM_FusBLPathC1Calc : Subsystem
  LM_FusBLPathC2Calc : Subsystem
  LM_FusBLPathC3Calc : Subsystem
  LM_FusBLPathQualityCalc : Stateflow chart  TreatAsAtomicUnit=on
  LM_FusBLPathC0 : Outport
  LM_FusBLPathC1 : Outport  Port=2
  LM_FusBLPathC2 : Outport  Port=3
  LM_FusBLPathC3 : Outport  Port=4
  LM_FusBLPathQuality : Outport  Port=5
  wires:
  [LM_FusBLPathQuality] -> LM_FusBLPathC3Calc/1(LM_FusBLPathQuality), LM_FusBLPathC2Calc/1(LM_FusBLPathQuality), LM_FusBLPathC1Calc/1(LM_FusBLPathQuality), LM_FusBLPathC0Calc/1(LM_FusBLPathQuality)
  LM_VSLFntPathP/1 -> LM_FusBLPathC3Calc/2(LM_VSLPathP), LM_FusBLPathC2Calc/2(LM_VSLPathP), LM_FusBLPathC1Calc/2(LM_VSLPathP), LM_FusBLPathC0Calc/2(LM_VSLPathP)
  LM_EMLFntPathP/1 -> LM_FusBLPathC0Calc/3(LM_EMLPathP), LM_FusBLPathC3Calc/3(LM_EMLPathP), LM_FusBLPathC2Calc/3(LM_EMLPathP), LM_FusBLPathC1Calc/3(LM_EMLPathP)
  LM_OTLFntPathP/1 -> LM_FusBLPathC0Calc/4(LM_OTLPathP), LM_FusBLPathC3Calc/4(LM_OTLPathP), LM_FusBLPathC2Calc/4(LM_OTLPathP), LM_FusBLPathC1Calc/4(LM_OTLPathP)
  LM_FusPathEMLK/1 -> LM_FusBLPathQualityCalc/4(LM_FusPathEMLK), LM_FusBLPathC0Calc/5(LM_FusPathEMLK), LM_FusBLPathC1Calc/5(LM_FusPathEMLK), LM_FusBLPathC2Calc/5(LM_FusPathEMLK), LM_FusBLPathC3Calc/5(LM_FusPathEMLK)
  LM_FusPathVSLK/1 -> LM_FusBLPathQualityCalc/5(LM_FusPathVSLK), LM_FusBLPathC0Calc/6(LM_FusPathVSLK), LM_FusBLPathC1Calc/6(LM_FusPathVSLK), LM_FusBLPathC2Calc/6(LM_FusPathVSLK), LM_FusBLPathC3Calc/6(LM_FusPathVSLK)
  LM_FusPathOTLK/1 -> LM_FusBLPathQualityCalc/6(LM_FusPathOTLK), LM_FusBLPathC0Calc/7(LM_FusPathOTLK), LM_FusBLPathC1Calc/7(LM_FusPathOTLK), LM_FusBLPathC2Calc/7(LM_FusPathOTLK), LM_FusBLPathC3Calc/7(LM_FusPathOTLK)
  LM_VSLPathQuality/1 -> LM_FusBLPathQualityCalc/2(LM_VSLPathQuality)
  LM_EMLPathQuality/1 -> LM_FusBLPathQualityCalc/1(LM_EMLPathQuality)
  LM_OTLPathQuality/1 -> LM_FusBLPathQualityCalc/3(LM_OTLPathQuality)
  LM_FusBLPathC0Calc/1(LM_FusBLPathC0) -> LM_FusBLPathC0/1
  LM_FusBLPathC1Calc/1(LM_FusBLPathC1) -> LM_FusBLPathC1/1
  LM_FusBLPathC2Calc/1(LM_FusBLPathC2) -> LM_FusBLPathC2/1
  LM_FusBLPathC3Calc/1(LM_FusBLPathC3) -> LM_FusBLPathC3/1
  LM_FusBLPathQualityCalc/1(LM_FusBLPathQuality) -> [LM_FusBLPathQuality], LM_FusBLPathQuality/1

== system PubIfDecisionLM_MDL/Subsystem2/LM_Fusion1/LM_FusBaseLineInfoCalc/LM_FusBLFntPath1130/LM_EVOFFntPath3 ==
  LM_VSLFntPathP : Inport
  LM_VSLPathQuality : Inport  Port=2
  LM_EMLFntPathP : Inport  Port=3
  LM_EMLPathQuality : Inport  Port=4
  LM_OTLFntPathP : Inport  Port=5
  LM_OTLPathQuality : Inport  Port=6
  LM_FusPathEMLK : Inport  Port=7
  LM_FusPathVSLK : Inport  Port=8
  LM_FusPathOTLK : Inport  Port=9
  LM_FusBLPathC0Calc : Subsystem
  LM_FusBLPathC1Calc : Subsystem
  LM_FusBLPathC2Calc : Subsystem
  LM_FusBLPathC3Calc : Subsystem
  LM_FusBLPathQualityCalc : Stateflow chart  TreatAsAtomicUnit=on
  LM_FusBLPathC0 : Outport
  LM_FusBLPathC1 : Outport  Port=2
  LM_FusBLPathC2 : Outport  Port=3
  LM_FusBLPathC3 : Outport  Port=4
  LM_FusBLPathQuality : Outport  Port=5
  wires:
  [LM_FusBLPathQuality] -> LM_FusBLPathC3Calc/1(LM_FusBLPathQuality), LM_FusBLPathC2Calc/1(LM_FusBLPathQuality), LM_FusBLPathC1Calc/1(LM_FusBLPathQuality), LM_FusBLPathC0Calc/1(LM_FusBLPathQuality)
  LM_VSLFntPathP/1 -> LM_FusBLPathC3Calc/2(LM_VSLPathP), LM_FusBLPathC2Calc/2(LM_VSLPathP), LM_FusBLPathC1Calc/2(LM_VSLPathP), LM_FusBLPathC0Calc/2(LM_VSLPathP)
  LM_EMLFntPathP/1 -> LM_FusBLPathC0Calc/3(LM_EMLPathP), LM_FusBLPathC3Calc/3(LM_EMLPathP), LM_FusBLPathC2Calc/3(LM_EMLPathP), LM_FusBLPathC1Calc/3(LM_EMLPathP)
  LM_OTLFntPathP/1 -> LM_FusBLPathC0Calc/4(LM_OTLPathP), LM_FusBLPathC3Calc/4(LM_OTLPathP), LM_FusBLPathC2Calc/4(LM_OTLPathP), LM_FusBLPathC1Calc/4(LM_OTLPathP)
  LM_FusPathEMLK/1 -> LM_FusBLPathQualityCalc/4(LM_FusPathEMLK), LM_FusBLPathC0Calc/5(LM_FusPathEMLK), LM_FusBLPathC1Calc/5(LM_FusPathEMLK), LM_FusBLPathC2Calc/5(LM_FusPathEMLK), LM_FusBLPathC3Calc/5(LM_FusPathEMLK)
  LM_FusPathVSLK/1 -> LM_FusBLPathQualityCalc/5(LM_FusPathVSLK), LM_FusBLPathC0Calc/6(LM_FusPathVSLK), LM_FusBLPathC1Calc/6(LM_FusPathVSLK), LM_FusBLPathC2Calc/6(LM_FusPathVSLK), LM_FusBLPathC3Calc/6(LM_FusPathVSLK)
  LM_FusPathOTLK/1 -> LM_FusBLPathQualityCalc/6(LM_FusPathOTLK), LM_FusBLPathC0Calc/7(LM_FusPathOTLK), LM_FusBLPathC1Calc/7(LM_FusPathOTLK), LM_FusBLPathC2Calc/7(LM_FusPathOTLK), LM_FusBLPathC3Calc/7(LM_FusPathOTLK)
  LM_VSLPathQuality/1 -> LM_FusBLPathQualityCalc/2(LM_VSLPathQuality)
  LM_EMLPathQuality/1 -> LM_FusBLPathQualityCalc/1(LM_EMLPathQuality)
  LM_OTLPathQuality/1 -> LM_FusBLPathQualityCalc/3(LM_OTLPathQuality)
  LM_FusBLPathC0Calc/1(LM_FusBLPathC0) -> LM_FusBLPathC0/1
  LM_FusBLPathC1Calc/1(LM_FusBLPathC1) -> LM_FusBLPathC1/1
  LM_FusBLPathC2Calc/1(LM_FusBLPathC2) -> LM_FusBLPathC2/1
  LM_FusBLPathC3Calc/1(LM_FusBLPathC3) -> LM_FusBLPathC3/1
  LM_FusBLPathQualityCalc/1(LM_FusBLPathQuality) -> [LM_FusBLPathQuality], LM_FusBLPathQuality/1

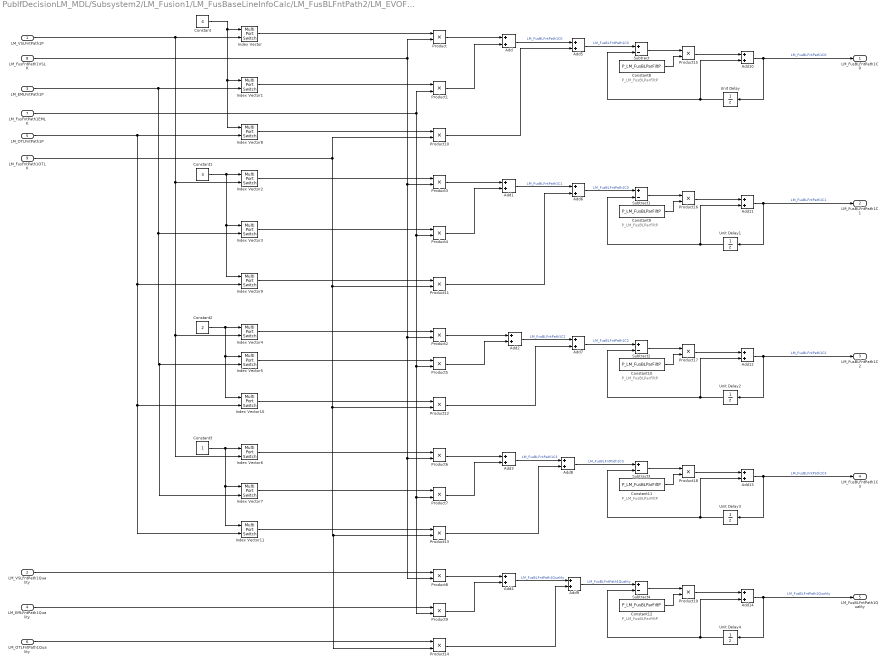
== system PubIfDecisionLM_MDL/Subsystem2/LM_Fusion1/LM_FusBaseLineInfoCalc/LM_FusBLFntPath2/LM_EVOFFntPath1 ==
  note: P_LM_FusBLParFiltP
  note: P_LM_FusBLParFiltP
  note: P_LM_FusBLParFiltP
  note: P_LM_FusBLParFiltP
  note: P_LM_FusBLParFiltP
  LM_VSLFntPath1P : Inport
  LM_VSLFntPath1Quality : Inport  Port=2
  LM_EMLFntPath1P : Inport  Port=3
  LM_EMLFntPath1Quality : Inport  Port=4
  LM_OTLFntPath1P : Inport  Port=5
  LM_OTLFntPath1Quality : Inport  Port=6
  LM_FusFntPath1EMLK : Inport  Port=7
  LM_FusFntPath1VSLK : Inport  Port=8
  LM_FusFntPath1OTLK : Inport  Port=9
  Add{,1..14} (15 alike) : Sum
  Constant : Constant  Value=4  OutDataTypeStr=uint8
  Constant1 : Constant  Value=3  OutDataTypeStr=uint8
  Constant{8..12} (5 alike) : Constant  Value=P_LM_FusBLParFiltP  OutDataTypeStr=single
  Constant2 : Constant  Value=2  OutDataTypeStr=uint8
  Constant3 : Constant  OutDataTypeStr=uint8
  Index Vector{,1..11} (12 alike) : MultiPortSwitch  Inputs=1
  Product{,1..19} (20 alike) : Product
  Subtract{,1..4} (5 alike) : Sum  Inputs=+-
  Unit Delay{,1..4} (5 alike) : UnitDelay  SampleTime=-1  HasFrameUpgradeWarning=on
  LM_FusBLFntPath1C0 : Outport
  LM_FusBLFntPath1C1 : Outport  Port=2
  LM_FusBLFntPath1C2 : Outport  Port=3
  LM_FusBLFntPath1C3 : Outport  Port=4
  LM_FusBLFntPath1Quality : Outport  Port=5
  wires:
  Add10/1 -> Unit Delay/1, LM_FusBLFntPath1C0/1  "LM_FusBLFntPath1C0"
  Add11/1 -> LM_FusBLFntPath1C1/1, Unit Delay1/1  "LM_FusBLFntPath1C1"
  Add12/1 -> LM_FusBLFntPath1C2/1, Unit Delay2/1  "LM_FusBLFntPath1C2"
  Product/1 -> Add/1
  Index Vector1/1 -> Product1/1
  Product1/1 -> Add/2
  Product4/1 -> Add1/2
  Index Vector3/1 -> Product4/1
  Product3/1 -> Add1/1
  Index Vector2/1 -> Product3/1
  Index Vector4/1 -> Product2/1
  LM_FusFntPath1VSLK/1 -> Product/2, Product2/2, Product8/2, Product6/2, Product3/2
  Product2/1 -> Add2/1
  Index Vector5/1 -> Product5/1
  LM_FusFntPath1EMLK/1 -> Product1/2, Product5/2, Product9/2, Product7/2, Product4/2
  Product5/1 -> Add2/2
  Index Vector/1 -> Product/1
  LM_EMLFntPath1P/1 -> Index Vector7/2, Index Vector5/2, Index Vector3/2, Index Vector1/2
  Index Vector6/1 -> Product6/1
  Index Vector7/1 -> Product7/1
  Product6/1 -> Add3/1
  Product7/1 -> Add3/2
  Add13/1 -> LM_FusBLFntPath1C3/1, Unit Delay3/1  "LM_FusBLFntPath1C3"
  LM_EMLFntPath1Quality/1 -> Product9/1
  Product8/1 -> Add4/1
  Product9/1 -> Add4/2
  Add14/1 -> LM_FusBLFntPath1Quality/1, Unit Delay4/1  "LM_FusBLFntPath1Quality"
  LM_VSLFntPath1P/1 -> Index Vector/2, Index Vector6/2, Index Vector4/2, Index Vector2/2
  LM_OTLFntPath1P/1 -> Index Vector11/2, Index Vector10/2, Index Vector9/2, Index Vector8/2
  Index Vector8/1 -> Product10/1
  LM_FusFntPath1OTLK/1 -> Product14/2, Product13/2, Product12/2, Product11/2, Product10/2
  Add/1 -> Add5/1  "LM_FusBLFntPath1C0"
  Product10/1 -> Add5/2
  Index Vector9/1 -> Product11/1
  Add1/1 -> Add6/1  "LM_FusBLFntPath1C1"
  Product11/1 -> Add6/2
  Index Vector10/1 -> Product12/1
  Add2/1 -> Add7/1  "LM_FusBLFntPath1C2"
  Product12/1 -> Add7/2
  Index Vector11/1 -> Product13/1
  Add3/1 -> Add8/1  "LM_FusBLFntPath1C3"
  Product13/1 -> Add8/2
  LM_OTLFntPath1Quality/1 -> Product14/1
  Add4/1 -> Add9/1  "LM_FusBLFntPath1Quality"
  Product14/1 -> Add9/2
  Constant/1 -> Index Vector1/1, Index Vector8/1, Index Vector/1
  Constant1/1 -> Index Vector3/1, Index Vector9/1, Index Vector2/1
  Constant2/1 -> Index Vector5/1, Index Vector10/1, Index Vector4/1
  Constant3/1 -> Index Vector7/1, Index Vector11/1, Index Vector6/1
  Add5/1 -> Subtract/1  "LM_FusBLFntPath1C0"
  Unit Delay/1 -> Add10/2, Subtract/2
  Product15/1 -> Add10/1
  Subtract/1 -> Product15/1
  Constant8/1 -> Product15/2
  Constant9/1 -> Product16/2
  Subtract1/1 -> Product16/1
  Product16/1 -> Add11/1
  Unit Delay1/1 -> Subtract1/2, Add11/2
  Add6/1 -> Subtract1/1  "LM_FusBLFntPath1C0"
  Unit Delay2/1 -> Add12/2, Subtract2/2
  Product17/1 -> Add12/1
  Subtract2/1 -> Product17/1
  Constant10/1 -> Product17/2
  Add7/1 -> Subtract2/1  "LM_FusBLFntPath1C2"
  Constant11/1 -> Product18/2
  Subtract3/1 -> Product18/1
  Product18/1 -> Add13/1
  Unit Delay3/1 -> Subtract3/2, Add13/2
  Add8/1 -> Subtract3/1  "LM_FusBLFntPath1C3"
  Unit Delay4/1 -> Add14/2, Subtract4/2
  Product19/1 -> Add14/1
  Subtract4/1 -> Product19/1
  Constant12/1 -> Product19/2
  Add9/1 -> Subtract4/1  "LM_FusBLFntPath1Quality"
  LM_VSLFntPath1Quality/1 -> Product8/1

== system PubIfDecisionLM_MDL/Subsystem2/LM_Fusion1/LM_FusBaseLineInfoCalc/LM_FusBLFntPath3/LM_EVOFFntPath1 ==
  LM_VSLFntPath1P : Inport
  LM_VSLFntPath1Quality : Inport  Port=2
  LM_EMLFntPath1P : Inport  Port=3
  LM_EMLFntPath1Quality : Inport  Port=4
  LM_OTLFntPath1P : Inport  Port=5
  LM_OTLFntPath1Quality : Inport  Port=6
  LM_FusFntPath1EMLK : Inport  Port=7
  LM_FusFntPath1VSLK : Inport  Port=8
  LM_FusFntPath1OTLK : Inport  Port=9
  Add{,1..9} (10 alike) : Sum
  Constant : Constant  Value=P_LM_FusParC0Index  OutDataTypeStr=uint8
  Constant1 : Constant  Value=P_LM_FusParC1Index  OutDataTypeStr=uint8
  Constant2 : Constant  Value=P_LM_FusParC2Index  OutDataTypeStr=uint8
  Constant3 : Constant  Value=P_LM_FusParC3Index  OutDataTypeStr=uint8
  Index Vector{,1..11} (12 alike) : MultiPortSwitch  Inputs=1
  Product{,1..14} (15 alike) : Product
  LM_FusBLFntPath1C0 : Outport
  LM_FusBLFntPath1C1 : Outport  Port=2
  LM_FusBLFntPath1C2 : Outport  Port=3
  LM_FusBLFntPath1C3 : Outport  Port=4
  LM_FusBLFntPath1Quality : Outport  Port=5
  wires:
  LM_VSLFntPath1Quality/1 -> Product8/1
  Add9/1 -> LM_FusBLFntPath1Quality/1  "LM_FusBLFntPath1Quality"
  Add8/1 -> LM_FusBLFntPath1C3/1  "LM_FusBLFntPath1C3"
  Add7/1 -> LM_FusBLFntPath1C2/1  "LM_FusBLFntPath1C2"
  Add6/1 -> LM_FusBLFntPath1C1/1  "LM_FusBLFntPath1C1"
  Add5/1 -> LM_FusBLFntPath1C0/1  "LM_FusBLFntPath1C0"
  Constant3/1 -> Index Vector6/1, Index Vector11/1, Index Vector7/1
  Constant2/1 -> Index Vector4/1, Index Vector10/1, Index Vector5/1
  Constant1/1 -> Index Vector2/1, Index Vector9/1, Index Vector3/1
  Constant/1 -> Index Vector/1, Index Vector8/1, Index Vector1/1
  Product14/1 -> Add9/2
  Add4/1 -> Add9/1  "LM_FusBLFntPath1Quality"
  LM_OTLFntPath1Quality/1 -> Product14/1
  Product13/1 -> Add8/2
  Add3/1 -> Add8/1  "LM_FusBLFntPath1C3"
  Index Vector11/1 -> Product13/1
  Product12/1 -> Add7/2
  Add2/1 -> Add7/1  "LM_FusBLFntPath1C2"
  Index Vector10/1 -> Product12/1
  Product11/1 -> Add6/2
  Add1/1 -> Add6/1  "LM_FusBLFntPath1C1"
  Index Vector9/1 -> Product11/1
  Product10/1 -> Add5/2
  Add/1 -> Add5/1  "LM_FusBLFntPath1C0"
  LM_FusFntPath1OTLK/1 -> Product10/2, Product11/2, Product12/2, Product13/2, Product14/2
  Index Vector8/1 -> Product10/1
  LM_OTLFntPath1P/1 -> Index Vector8/2, Index Vector9/2, Index Vector10/2, Index Vector11/2
  LM_VSLFntPath1P/1 -> Index Vector/2, Index Vector2/2, Index Vector4/2, Index Vector6/2
  Product9/1 -> Add4/2
  Product8/1 -> Add4/1
  LM_EMLFntPath1Quality/1 -> Product9/1
  Product7/1 -> Add3/2
  Product6/1 -> Add3/1
  Index Vector7/1 -> Product7/1
  Index Vector6/1 -> Product6/1
  LM_EMLFntPath1P/1 -> Index Vector1/2, Index Vector3/2, Index Vector5/2, Index Vector7/2
  Index Vector/1 -> Product/1
  Product5/1 -> Add2/2
  LM_FusFntPath1EMLK/1 -> Product4/2, Product7/2, Product9/2, Product5/2, Product1/2
  Index Vector5/1 -> Product5/1
  Product2/1 -> Add2/1
  LM_FusFntPath1VSLK/1 -> Product3/2, Product6/2, Product8/2, Product2/2, Product/2
  Index Vector4/1 -> Product2/1
  Index Vector2/1 -> Product3/1
  Product3/1 -> Add1/1
  Index Vector3/1 -> Product4/1
  Product4/1 -> Add1/2
  Product1/1 -> Add/2
  Index Vector1/1 -> Product1/1
  Product/1 -> Add/1

== system PubIfDecisionLM_MDL/Subsystem2/LM_Fusion1/LM_FusBaseLineInfoCalc/LM_FusBLRearPath/LM_EMLRearPath2 ==
  LM_VSLRearPath2P : Inport
  LM_VSLRearPath1Quality : Inport  Port=2
  Constant4 : Constant  Value=P_LM_FusParC0Index  OutDataTypeStr=uint8
  Constant5 : Constant  Value=P_LM_FusParC1Index  OutDataTypeStr=uint8
  Constant6 : Constant  Value=P_LM_FusParC3Index  OutDataTypeStr=uint8
  Constant7 : Constant  Value=P_LM_FusParC2Index  OutDataTypeStr=uint8
  Index Vector{,1..3} (4 alike) : MultiPortSwitch  Inputs=1
  Signal Conversion : SignalConversion  OverrideOpt=off
  LM_FusBLRearPath2C0 : Outport
  LM_FusBLRearPath2C1 : Outport  Port=2
  LM_FusBLRearPath2C2 : Outport  Port=3
  LM_FusBLRearPath2C3 : Outport  Port=4
  LM_FusBLRearPath2Quality : Outport  Port=5
  wires:
  LM_VSLRearPath1Quality/1 -> Signal Conversion/1
  LM_VSLRearPath2P/1 -> Index Vector/2, Index Vector1/2, Index Vector2/2, Index Vector3/2
  Constant7/1 -> Index Vector2/1
  Constant6/1 -> Index Vector3/1
  Constant5/1 -> Index Vector1/1
  Constant4/1 -> Index Vector/1
  Index Vector/1 -> LM_FusBLRearPath2C0/1  "LM_FusBLRearPath2C0"
  Index Vector1/1 -> LM_FusBLRearPath2C1/1  "LM_FusBLRearPath2C1"
  Index Vector2/1 -> LM_FusBLRearPath2C2/1  "LM_FusBLRearPath2C2"
  Index Vector3/1 -> LM_FusBLRearPath2C3/1  "LM_FusBLRearPath2C3"
  Signal Conversion/1 -> LM_FusBLRearPath2Quality/1  "LM_FusBLRearPath2Quality"

== system PubIfDecisionLM_MDL/Subsystem2/LM_Fusion1/LM_FusBaseLineInfoCalc/LM_FusBLRearPath/LM_EMLRearPath3 ==
  LM_VSLRearPath3P : Inport
  LM_VSLRearPath3Quality : Inport  Port=2
  Constant4 : Constant  Value=P_LM_FusParC0Index  OutDataTypeStr=uint8
  Constant5 : Constant  Value=P_LM_FusParC1Index  OutDataTypeStr=uint8
  Constant6 : Constant  Value=P_LM_FusParC3Index  OutDataTypeStr=uint8
  Constant7 : Constant  Value=P_LM_FusParC2Index  OutDataTypeStr=uint8
  Index Vector{,1..3} (4 alike) : MultiPortSwitch  Inputs=1
  Signal Conversion : SignalConversion  OverrideOpt=off
  LM_FusBLRearPath3C0 : Outport
  LM_FusBLRearPath3C1 : Outport  Port=2
  LM_FusBLRearPath3C2 : Outport  Port=3
  LM_FusBLRearPath3C3 : Outport  Port=4
  LM_FusBLRearPath3Quality : Outport  Port=5
  wires:
  LM_VSLRearPath3Quality/1 -> Signal Conversion/1
  LM_VSLRearPath3P/1 -> Index Vector/2, Index Vector1/2, Index Vector2/2, Index Vector3/2
  Constant7/1 -> Index Vector2/1
  Constant6/1 -> Index Vector3/1
  Constant5/1 -> Index Vector1/1
  Constant4/1 -> Index Vector/1
  Index Vector/1 -> LM_FusBLRearPath3C0/1  "LM_FusBLRearPath3C0"
  Index Vector1/1 -> LM_FusBLRearPath3C1/1  "LM_FusBLRearPath3C1"
  Index Vector2/1 -> LM_FusBLRearPath3C2/1  "LM_FusBLRearPath3C2"
  Index Vector3/1 -> LM_FusBLRearPath3C3/1  "LM_FusBLRearPath3C3"
  Signal Conversion/1 -> LM_FusBLRearPath3Quality/1  "LM_FusBLRearPath3Quality"

== system PubIfDecisionLM_MDL/Subsystem2/LM_Fusion1/LM_FusBaseLineInfoCalc/LM_FusBLRearPath/LM_EMLRearPath4 ==
  LM_VSLRearPath1P : Inport
  LM_VSLRearPath1Quality : Inport  Port=2
  Constant : Constant  Value=P_LM_FusParC0Index  OutDataTypeStr=uint8
  Constant1 : Constant  Value=P_LM_FusParC1Index  OutDataTypeStr=uint8
  Constant2 : Constant  Value=P_LM_FusParC3Index  OutDataTypeStr=uint8
  Constant4 : Constant  Value=P_LM_FusParC2Index  OutDataTypeStr=uint8
  Index Vector{,1..3} (4 alike) : MultiPortSwitch  Inputs=1
  Signal Conversion : SignalConversion  OverrideOpt=off
  LM_FusBLRearPath1C0 : Outport
  LM_FusBLRearPath1C1 : Outport  Port=2
  LM_FusBLRearPath1C2 : Outport  Port=3
  LM_FusBLRearPath1C3 : Outport  Port=4
  LM_FusBLRearPath1Quality : Outport  Port=5
  wires:
  Constant/1 -> Index Vector/1
  Constant1/1 -> Index Vector1/1
  Constant2/1 -> Index Vector3/1
  Constant4/1 -> Index Vector2/1
  LM_VSLRearPath1P/1 -> Index Vector/2, Index Vector1/2, Index Vector2/2, Index Vector3/2
  LM_VSLRearPath1Quality/1 -> Signal Conversion/1
  Index Vector/1 -> LM_FusBLRearPath1C0/1  "LM_FusBLRearPath1C0"
  Index Vector1/1 -> LM_FusBLRearPath1C1/1  "LM_FusBLRearPath1C1"
  Index Vector2/1 -> LM_FusBLRearPath1C2/1  "LM_FusBLRearPath1C2"
  Index Vector3/1 -> LM_FusBLRearPath1C3/1  "LM_FusBLRearPath1C3"
  Signal Conversion/1 -> LM_FusBLRearPath1Quality/1  "LM_FusBLRearPath1Quality"

== system PubIfDecisionLM_MDL/Subsystem2/LM_Fusion1/LM_FusRatioCalc/LM_FusionCase/LM_FusCaseJudge ==
  note: 0-EML
      | 1-VSL+EML
      | 2-VSL+EML+OTL
      | 3-EML+OTL
  LM_FusVSLValid : Inport
  LM_FusOTLValid : Inport  Port=2
  Constant1 : Constant  OutDataTypeStr=uint8
  Constant4 : Constant  Value=2  OutDataTypeStr=uint8
  Constant5 : Constant  Value=0  OutDataTypeStr=uint8
  Constant6 : Constant  Value=3  OutDataTypeStr=uint8
  Logical Operator : Logic  AllPortsSameDT=off  OutDataTypeStr=boolean
  Logical Operator1 : Logic  AllPortsSameDT=off  OutDataTypeStr=boolean
  Logical Operator2 : Logic  Operator=NOT  AllPortsSameDT=off  OutDataTypeStr=boolean
  Logical Operator3 : Logic  AllPortsSameDT=off  OutDataTypeStr=boolean
  Logical Operator4 : Logic  Operator=NOT  AllPortsSameDT=off  OutDataTypeStr=boolean
  Switch : Switch  Criteria=u2 ~= 0
  Switch1 : Switch  Criteria=u2 ~= 0
  Switch2 : Switch  Criteria=u2 ~= 0
  LM_FusCase : Outport
  wires:
  Logical Operator/1 -> Switch1/2
  Switch1/1 -> LM_FusCase/1  "LM_FusCase"
  Constant4/1 -> Switch1/1
  Logical Operator2/1 -> Logical Operator1/1
  Logical Operator3/1 -> Switch/2
  Logical Operator1/1 -> Switch2/2
  Logical Operator4/1 -> Logical Operator3/2
  Switch/1 -> Switch2/3  "LM_FusionCase"
  Constant5/1 -> Switch/3
  LM_FusVSLValid/1 -> Logical Operator3/1, Logical Operator2/1, Logical Operator/1
  Constant6/1 -> Switch2/1
  Constant1/1 -> Switch/1
  LM_FusOTLValid/1 -> Logical Operator4/1, Logical Operator1/2, Logical Operator/2
  Switch2/1 -> Switch1/3

== system PubIfDecisionLM_MDL/Subsystem2/LM_Fusion1/LM_FusRatioCalc/LM_FusionCase/LM_FusCaseOTLValidJudge ==
  note: P_LM_FusOTLQuaThre
  note: P_LM_FusOTLSW
  LM_OTLFntPath1Qulity : Inport
  LM_OTLFntPath2Qulity : Inport  Port=2
  LM_OTLFntPath3Qulity : Inport  Port=3
  Compare To Constant1 : simulink/Logic and Bit Operations/Compare To Constant  relop===  const=1  OutDataTypeStr=boolean
  Constant3 : Constant  Value=P_LM_FusOTLQuaThre
  Constant7 : Constant  Value=P_LM_FusOTLSW  OutDataTypeStr=uint8
  Logical Operator6 : Logic  AllPortsSameDT=off  OutDataTypeStr=boolean
  Max : MinMax  Function=max  Inputs=3
  Relational Operator1 : RelationalOperator  OutDataTypeStr=boolean  RndMeth=Nearest
  LM_FusOTLValid : Outport
  wires:
  Compare To Constant1/1 -> Logical Operator6/1
  Max/1 -> Relational Operator1/1
  LM_OTLFntPath2Qulity/1 -> Max/2
  Relational Operator1/1 -> Logical Operator6/2
  Constant3/1 -> Relational Operator1/2
  Constant7/1 -> Compare To Constant1/1
  Logical Operator6/1 -> LM_FusOTLValid/1  "LM_FusOTLValid"
  LM_OTLFntPath1Qulity/1 -> Max/1
  LM_OTLFntPath3Qulity/1 -> Max/3

== system PubIfDecisionLM_MDL/Subsystem2/LM_Fusion1/LM_FusRatioCalc/LM_FusionCase/LM_FusCaseVSLValidJudge ==
  note: 0.1
  note: P_LM_FusVSLSW
  LM_VSLFntPaht1Quality : Inport
  vxvRefMs : Inport  Port=2
  SteerWheelAng : Inport  Port=3
  Compare To Constant : simulink/Logic and Bit Operations/Compare To Constant  relop===  const=1  OutDataTypeStr=boolean
  Constant : Constant  Value=P_LM_FusVSLQuaThre  OutDataTypeStr=single
  Constant2 : Constant  Value=P_LM_FusVSLSW  OutDataTypeStr=uint8
  Constant8 : Constant  Value=P_LM_FusVSLValidVxvThre  OutDataTypeStr=single
  Constant9 : Constant  Value=P_LM_FusVSLValidSteerWheerAngThre  OutDataTypeStr=single
  Logical Operator5 : Logic  Inputs=3  AllPortsSameDT=off  OutDataTypeStr=boolean
  Logical Operator7 : Logic  AllPortsSameDT=off  OutDataTypeStr=boolean
  Logical Operator8 : Logic  Operator=NOT  AllPortsSameDT=off  OutDataTypeStr=boolean
  Relational Operator : RelationalOperator  OutDataTypeStr=boolean  RndMeth=Nearest
  Relational Operator2 : RelationalOperator  Operator=<=  OutDataTypeStr=boolean  RndMeth=Simplest
  Relational Operator3 : RelationalOperator  OutDataTypeStr=boolean  RndMeth=Simplest
  LM_FusVSLValid : Outport
  wires:
  Logical Operator7/1 -> Logical Operator8/1
  Relational Operator3/1 -> Logical Operator7/2
  Constant9/1 -> Relational Operator3/2
  SteerWheelAng/1 -> Relational Operator3/1
  Relational Operator/1 -> Logical Operator5/2
  Constant/1 -> Relational Operator/2
  vxvRefMs/1 -> Relational Operator2/1
  Constant2/1 -> Compare To Constant/1
  Logical Operator5/1 -> LM_FusVSLValid/1  "LM_FusVSLValid"
  Logical Operator8/1 -> Logical Operator5/3
  Relational Operator2/1 -> Logical Operator7/1
  Constant8/1 -> Relational Operator2/2
  LM_VSLFntPaht1Quality/1 -> Relational Operator/1
  Compare To Constant/1 -> Logical Operator5/1

== system PubIfDecisionLM_MDL/Subsystem2/LM_Fusion1/LM_FusRatioCalc/LM_Fusion_EMLOnly/LM_FusBaseLineC0Info ==
  LM_EMLLLC0 : Inport
  LM_EMLC0 : Inport  Port=2
  LM_EMLRLC0 : Inport  Port=3
  LM_EMLRRC0 : Inport  Port=4
  Signal Conversion{,1..3} (4 alike) : SignalConversion  OverrideOpt=off
  LM_LLC0 : Outport
  LM_LRC0 : Outport  Port=2
  LM_RLC0 : Outport  Port=3
  LM_RRC0 : Outport  Port=4
  wires:
  LM_EMLLLC0/1 -> Signal Conversion/1
  LM_EMLC0/1 -> Signal Conversion1/1
  LM_EMLRLC0/1 -> Signal Conversion2/1
  LM_EMLRRC0/1 -> Signal Conversion3/1
  Signal Conversion/1 -> LM_LLC0/1  "LM_LLC0"
  Signal Conversion1/1 -> LM_LRC0/1  "LM_LRC0"
  Signal Conversion2/1 -> LM_RLC0/1  "LM_RLC0"
  Signal Conversion3/1 -> LM_RRC0/1  "LM_RRC0"
